simulink subsystem "hardware_hiding"  (R2024b)
settings: Solver=VariableStepAuto  StartTime=0.0  StopTime=10.0  RelTol=1e-3
undefined symbols (not defined in the file): D10, D11, D12, D2, D4, D5, D7, D8, D9, PTA0, PTA2, PTB23, PTB9, PTC3, PTC4, PTD0, PTD2, PTD3
libraries: frdmk64flib x10
settings Model: Creator=habel  LastModifiedBy=marwa

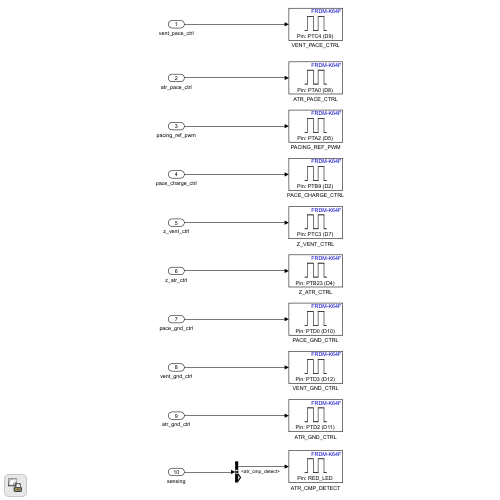
[thumbnail: Simulink's stored preview of the top-level diagram]
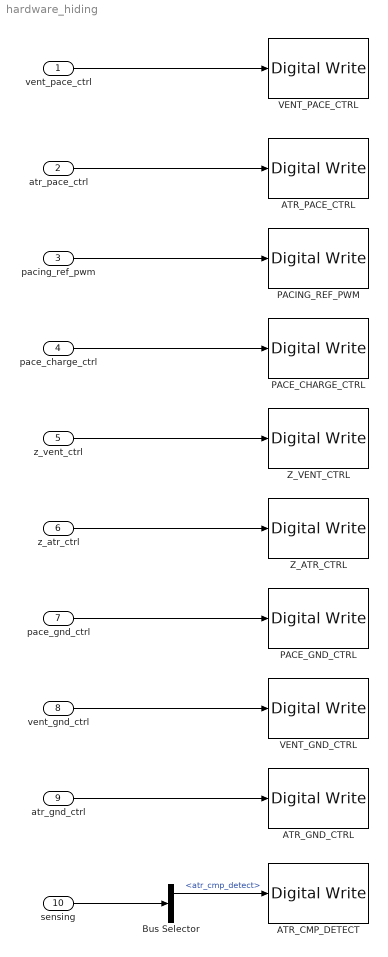
== system hardware_hiding ==
  vent_pace_ctrl : Inport
  atr_pace_ctrl : Inport  Port=2
  pacing_ref_pwm : Inport  Port=3
  pace_charge_ctrl : Inport  Port=4
  z_vent_ctrl : Inport  Port=5
  z_atr_ctrl : Inport  Port=6
  pace_gnd_ctrl : Inport  Port=7
  vent_gnd_ctrl : Inport  Port=8
  atr_gnd_ctrl : Inport  Port=9
  sensing : Inport  Port=10
  ATR_CMP_DETECT : frdmk64flib/Digital Write  Whichpin=RED_LED
  ATR_GND_CTRL : frdmk64flib/Digital Write  Whichpin=PTD2 (D11)
  ATR_PACE_CTRL : frdmk64flib/Digital Write  Whichpin=PTA0 (D8)
  Bus Selector : BusSelector  OutputSignals=atr_cmp_detect,vent_cmp_detect
  PACE_CHARGE_CTRL : frdmk64flib/Digital Write  Whichpin=PTB9 (D2)
  PACE_GND_CTRL : frdmk64flib/Digital Write  Whichpin=PTD0 (D10)
  PACING_REF_PWM : frdmk64flib/Digital Write  Whichpin=PTA2 (D5)
  VENT_GND_CTRL : frdmk64flib/Digital Write  Whichpin=PTD3 (D12)
  VENT_PACE_CTRL : frdmk64flib/Digital Write  Whichpin=PTC4 (D9)
  Z_ATR_CTRL : frdmk64flib/Digital Write  Whichpin=PTB23 (D4)
  Z_VENT_CTRL : frdmk64flib/Digital Write  Whichpin=PTC3 (D7)
  wires:
  z_atr_ctrl/1 -> Z_ATR_CTRL/1
  vent_pace_ctrl/1 -> VENT_PACE_CTRL/1
  vent_gnd_ctrl/1 -> VENT_GND_CTRL/1
  pacing_ref_pwm/1 -> PACING_REF_PWM/1
  atr_pace_ctrl/1 -> ATR_PACE_CTRL/1
  pace_charge_ctrl/1 -> PACE_CHARGE_CTRL/1
  pace_gnd_ctrl/1 -> PACE_GND_CTRL/1
  atr_gnd_ctrl/1 -> ATR_GND_CTRL/1
  z_vent_ctrl/1 -> Z_VENT_CTRL/1
  sensing/1 -> Bus Selector/1
  Bus Selector/1 -> ATR_CMP_DETECT/1  "<atr_cmp_detect>"
